simulink model "MotorEstimation_R2019a"  (R2023a)
settings: Solver=VariableStepAuto  StartTime=0.0  StopTime=30  MaxStep=0.01  RelTol=1e-3
InitFcn:
  | JointParameters
values from neighbouring files (symbols this model uses):
  a = 0    [JointParameters.m]
  a1 = 0    [JointParameters.m]
  a2 = 0    [JointParameters.m]
  b = 1    [JointParameters.m]
  b1 = 1    [JointParameters.m]
  b2 = 1    [JointParameters.m]
  B_l = 0    [JointParameters.m]
  B_u = 0    [JointParameters.m]
  g = 9.81    [JointParameters.m]
  J_l = 0.071440709    [JointParameters.m]
  J_u = 0.049103    [JointParameters.m]
  k = 0.32    [JointParameters.m]
  k1 = 0.2    [JointParameters.m]
  k2 = 0.2    [JointParameters.m]
  L_cg_l = 0.102366    [JointParameters.m]
  L_cg_u = 0.066301    [JointParameters.m]
  L_l = 0.223793    [JointParameters.m]
  L_u = 0.227293    [JointParameters.m]
  mass_l = 2.495    [JointParameters.m]
  mass_u = 2.024    [JointParameters.m]
settings Model: Creator=user  LastModifiedBy=user

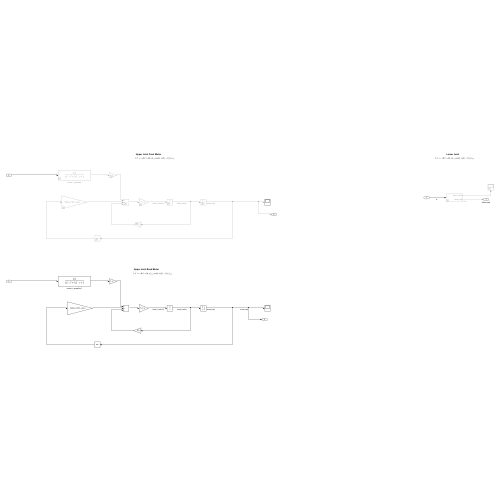
[thumbnail: Simulink's stored preview of the top-level diagram]
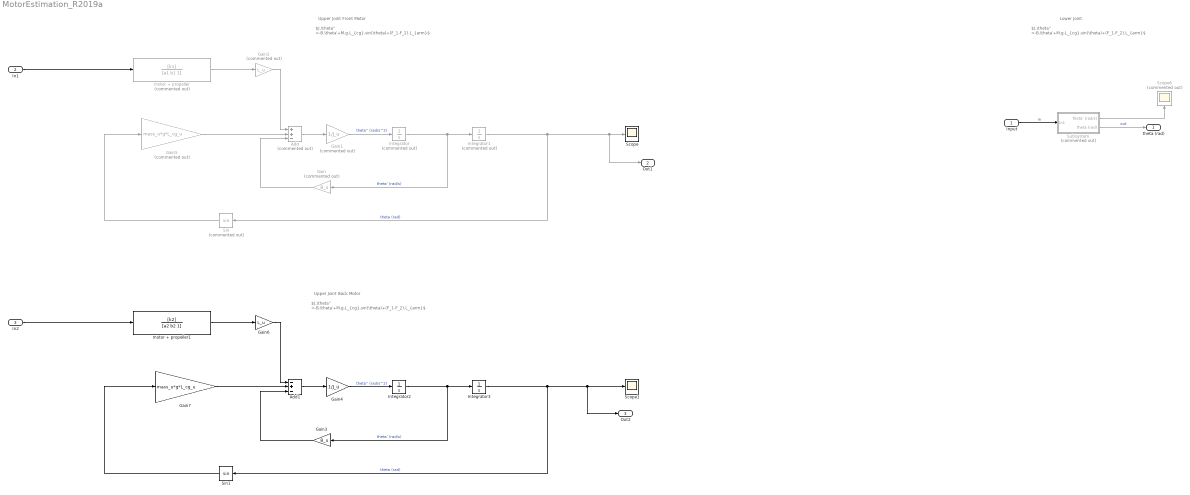
== system MotorEstimation_R2019a ==
  note: $J.\theta'' =-B.\theta'+M.g.L_{cg}.sin(\theta)+(F_1-F_2).L_{arm}$
  note: Upper Joint Front Motor
  note: $J.\theta'' =-B.\theta'+M.g.L_{cg}.sin(\theta)+(F_1-F_2).L_{arm}$
  note: Lower Joint
  note: $J.\theta'' =-B.\theta'+M.g.L_{cg}.sin(\theta)+(F_1-F_2).L_{arm}$
  note: Upper Joint Back Motor
  Input : Inport
  In1 : Inport  Port=2
  In2 : Inport  Port=3
  Add : Sum  Commented=on  Inputs=++-
  Add1 : Sum  Inputs=-+-
  Gain : Gain  Commented=on  Gain=B_u
  Gain1 : Gain  Commented=on  Gain=1/J_u
  Gain2 : Gain  Commented=on  Gain=L_u
  Gain3 : Gain  Gain=B_u
  Gain4 : Gain  Gain=1/J_u
  Gain5 : Gain  Commented=on  Gain=mass_u*g*L_cg_u
  Gain6 : Gain  Gain=L_u
  Gain7 : Gain  Gain=mass_u*g*L_cg_u
  Integrator : Integrator  Commented=on
  Integrator1 : Integrator  Commented=on  InitialCondition=-0.33  LimitOutput=on  UpperSaturationLimit=.4  LowerSaturationLimit=-.33
  Integrator2 : Integrator
  Integrator3 : Integrator  InitialCondition=0.4  LimitOutput=on  UpperSaturationLimit=.4  LowerSaturationLimit=-.33
  Scope : Scope
  Scope1 : Scope
  Scope6 : Scope  Commented=on
  Sin : Trigonometry  Commented=on
  Sin1 : Trigonometry
  Subsystem : Subsystem  Commented=on
  motor + propeller : TransferFcn  Commented=on  Numerator=[k1]  Denominator=[a1 b1 1]
  motor + propeller1 : TransferFcn  Numerator=[k2]  Denominator=[a2 b2 1]
  theta (rad) : Outport
  Out1 : Outport  Port=2
  Out2 : Outport  Port=3
  wires:
  Gain1/1 -> Integrator/1  "theta'' (rad/s^2)"
  Integrator/1 -> Gain/1, Integrator1/1  "theta' (rad/s)"
  Integrator1/1 -> Out1/1, Scope/1, Sin/1  "theta (rad)"
  motor + propeller/1 -> Gain2/1
  Sin/1 -> Gain5/1
  Gain5/1 -> Add/2
  Gain/1 -> Add/3
  Add/1 -> Gain1/1
  Gain2/1 -> Add/1
  In1/1 -> motor + propeller/1
  Input/1 -> Subsystem/1(In1)  "in"
  Subsystem/1(theta' (rad/s)) -> Scope6/1
  Subsystem/2(theta (rad)) -> theta (rad)/1  "out"
  In2/1 -> motor + propeller1/1
  Gain6/1 -> Add1/1
  Add1/1 -> Gain4/1
  Gain3/1 -> Add1/3
  Gain7/1 -> Add1/2
  Sin1/1 -> Gain7/1
  motor + propeller1/1 -> Gain6/1
  Integrator2/1 -> Integrator3/1, Gain3/1  "theta' (rad/s)"
  Gain4/1 -> Integrator2/1  "theta'' (rad/s^2)"
  Integrator3/1 -> Sin1/1, Out2/1, Scope1/1  "theta (rad)"

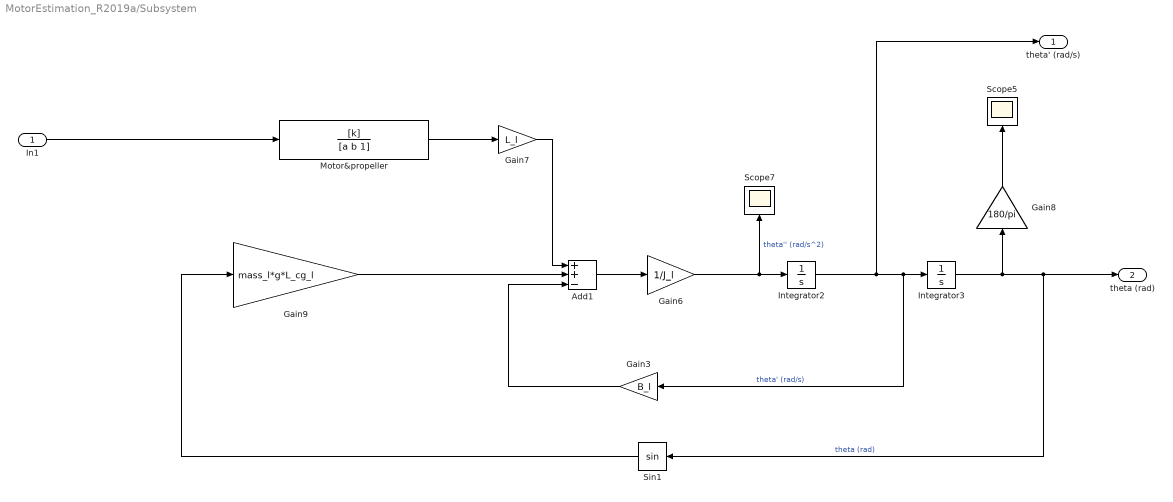
== system MotorEstimation_R2019a/Subsystem ==
  In1 : Inport
  Add1 : Sum  Inputs=++-
  Gain3 : Gain  Gain=B_l
  Gain6 : Gain  Gain=1/J_l
  Gain7 : Gain  Gain=L_l
  Gain8 : Gain  Gain=180/pi
  Gain9 : Gain  Gain=mass_l*g*L_cg_l
  Integrator2 : Integrator
  Integrator3 : Integrator  InitialCondition=-0.33  LimitOutput=on  UpperSaturationLimit=0.4  LowerSaturationLimit=-0.33
  Motor&propeller : TransferFcn  Numerator=[k]  Denominator=[a b 1]
  Scope5 : Scope
  Scope7 : Scope
  Sin1 : Trigonometry
  theta' (rad/s) : Outport
  theta (rad) : Outport  Port=2
  wires:
  Gain3/1 -> Add1/3
  Integrator3/1 -> Gain8/1, theta (rad)/1, Sin1/1  "theta (rad)"
  Sin1/1 -> Gain9/1
  Motor&propeller/1 -> Gain7/1
  Add1/1 -> Gain6/1
  Gain7/1 -> Add1/1
  Gain8/1 -> Scope5/1
  Gain9/1 -> Add1/2
  Integrator2/1 -> theta' (rad/s)/1, Integrator3/1, Gain3/1  "theta' (rad/s)"
  Gain6/1 -> Integrator2/1, Scope7/1  "theta'' (rad/s^2)"
  In1/1 -> Motor&propeller/1
